simulink model "filter_high_pass"  (R2020a)
settings: Solver=FixedStepAuto  StartTime=0.0  StopTime=10  RelTol=1e-3
settings Model: Creator=sadamu  LastModifiedBy=sadamu
settings SolverCC: AutoInsertRateTranBlk=on
settings DataIOCC: LimitDataPoints=on  SaveOutput=off  SignalLogging=off  DSMLogging=off  SaveTime=off
settings OptimizationCC: DefaultParameterBehavior=Inlined  DefaultUnderspecifiedDataType=single  StrengthReduction=on  PassReuseOutputArgsAs=Individual arguments  ZeroExternalMemoryAtStartup=off  ZeroInternalMemoryAtStartup=off  OptimizeBlockOrder=speed  OptimizationPriority=Speed  OptimizationCustomize=off  MultiThreadedLoops=on  EfficientTunableParamExpr=on
settings DebuggingCC: AlgebraicLoopMsg=error  SingleTaskRateTransMsg=error  ParameterTunabilityLossMsg=error  AllowSymbolicDim=off  SFUnexpectedBacktrackingDiag=warning  SFNoUnconditionalDefaultTransitionDiag=warning  SFExecutionAtInitializationDiag=none  ArithmeticOperatorsInVariantConditions=warning
settings HardwareCC: ProdBitPerPointer=32  ProdBitPerSizeT=32  ProdBitPerPtrDiffT=32  ProdLargestAtomicInteger=Long  ProdLargestAtomicFloat=Double  ProdWordSize=32  ProdHWDeviceType=ARM Compatible->ARM Cortex
settings SFSimCC: SimUseLocalCustomCode=off  MATLABDynamicMemAlloc=off  CustomCodeUndefinedFunction=UseInterfaceOnly
settings RTWCC: SystemTargetFile=ert.tlc  GenCodeOnly=on  TemplateMakefile=ert_default_tmf  GenerateReport=on  RTWUseLocalCustomCode=off  BuildConfiguration=Debug  LaunchReport=on
settings CodeAppCC: GenerateComments=off  IgnoreCustomStorageClasses=off  OperatorAnnotations=on  SimulinkDataObjDesc=on  SFDataObjDesc=on  InsertBlockDesc=on  EnableCustomComments=on
settings ERTTargetCC: CodeReplacementLibrary=Inlined ARM NEON Intrinsics  GenerateSampleERTMain=on  InlinedParameterPlacement=NonHierarchical  ERTCustomFileTemplate=example_file_process.tlc

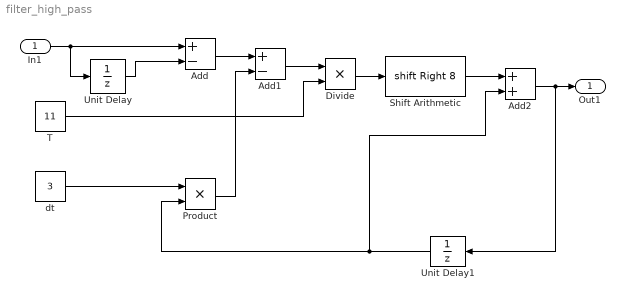
== system filter_high_pass ==
  In1 : Inport  OutDataTypeStr=int32  PortDimensions=32
  Add : Sum  Inputs=+-
  Add1 : Sum  Inputs=+-
  Add2 : Sum
  Divide : Product  Inputs=**  OutDataTypeStr=int32
  Product : Product  OutDataTypeStr=int32
  Shift Arithmetic : ArithShift  BitShiftNumber=8  BitShiftDirection=Right
  T : Constant  Value=11  OutDataTypeStr=int32  SampleTime=0.1
  Unit Delay : UnitDelay  SampleTime=-1  HasFrameUpgradeWarning=on
  Unit Delay1 : UnitDelay  SampleTime=-1  HasFrameUpgradeWarning=on
  dt : Constant  Value=3  OutDataTypeStr=int32  SampleTime=0.1
  Out1 : Outport
  wires:
  Add/1 -> Add1/1
  Add1/1 -> Divide/1
  Add2/1 -> Unit Delay1/1, Out1/1
  dt/1 -> Product/1
  Divide/1 -> Shift Arithmetic/1
  In1/1 -> Add/1, Unit Delay/1
  T/1 -> Divide/2
  Unit Delay/1 -> Add/2
  Unit Delay1/1 -> Product/2, Add2/2
  Product/1 -> Add1/2
  Shift Arithmetic/1 -> Add2/1
